simulink library "xrbsDSP_r4"  (Simulink 7.1)
undefined symbols (not defined in the file or in its folder): mem
libraries: xbsIndex_r4 x330
(part 3 of 5)

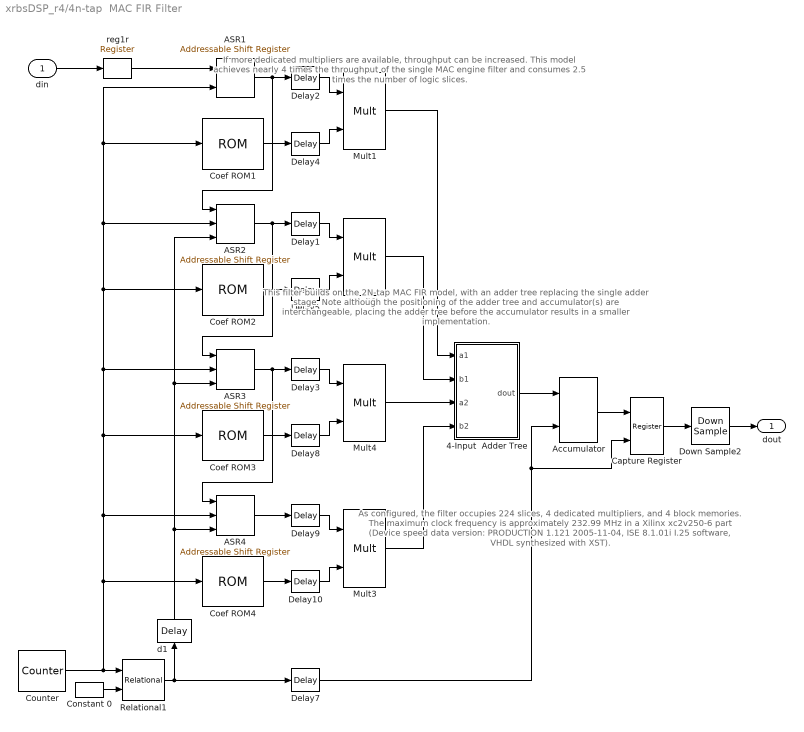
== system xrbsDSP_r4/4n-tap  MAC FIR Filter ==
  note: This filter builds on the 2N-tap MAC FIR model, with an adder tree
      | replacing the single adder stage.  Note although the positioning
      | of the adder tree and accumulator(s) are interchangeable, placing
      | the adder tree before the accumulator results in a smaller
      | implementation.
  note: As configured, the filter occupies 224 slices, 4 dedicated multipliers,
      | and 4 block memories.  The maximum clock frequency is approximately
      |  232.99 MHz in a Xilinx xc2v250-6 part (Device speed data version:
      | PRODUCTION 1.121 2005-11-04, ISE 8.1.01i I.25 software, VHDL
      | synthesized with XST).
  note: If more dedicated multipliers are available, throughput
      | can be increased.  This model achieves nearly 4 times
      | the throughput of the single MAC engine filter and
      | consumes 2.5 times the number of logic slices.
  din : Inport  OutDataType=sfix(16)  OutScaling=2^0
  4-Input  Adder Tree : Subsystem
  ASR1 : xbsIndex_r4/Addressable Shift Register  infer_latency=on  depth=2  initVector=0  en=off  dbl_ovrd=off  use_behavioral_HDL=off  use_rpm=off  block_type=addrsr
      settings: infoedit="Delay of configurable length.  Any element in the delay line can be addressed and driven onto the output port.<P><P>Hardware notes: Implemented using SRL16s.  If a Virtex-II device is used, multiple SRLC16s are cascaded together."  xl_area=[0, 0, 0, 0, 0, 0, 0]  block_version=VER_STRING_GOES_HERE
  ASR2 : xbsIndex_r4/Addressable Shift Register  infer_latency=on  depth=2  initVector=0  en=on  dbl_ovrd=off  use_behavioral_HDL=off  use_rpm=off  block_type=addrsr
      settings: infoedit="Delay of configurable length.  Any element in the delay line can be addressed and driven onto the output port.<P><P>Hardware notes: Implemented using SRL16s.  If a Virtex-II device is used, multiple SRLC16s are cascaded together."  xl_area=[0, 0, 0, 0, 0, 0, 0]  block_version=VER_STRING_GOES_HERE
  ASR3 : xbsIndex_r4/Addressable Shift Register  infer_latency=on  depth=2  initVector=0  en=on  dbl_ovrd=off  use_behavioral_HDL=off  use_rpm=off  block_type=addrsr
      settings: infoedit="Delay of configurable length.  Any element in the delay line can be addressed and driven onto the output port.<P><P>Hardware notes: Implemented using SRL16s.  If a Virtex-II device is used, multiple SRLC16s are cascaded together."  xl_area=[0, 0, 0, 0, 0, 0, 0]  block_version=VER_STRING_GOES_HERE
  ASR4 : xbsIndex_r4/Addressable Shift Register  infer_latency=on  depth=2  initVector=0  en=on  dbl_ovrd=off  use_behavioral_HDL=off  use_rpm=off  block_type=addrsr
      settings: infoedit="Delay of configurable length.  Any element in the delay line can be addressed and driven onto the output port.<P><P>Hardware notes: Implemented using SRL16s.  If a Virtex-II device is used, multiple SRLC16s are cascaded together."  xl_area=[0, 0, 0, 0, 0, 0, 0]  block_version=VER_STRING_GOES_HERE
  Accumulator : xbsIndex_r4/Accumulator  operation=Add  n_bits=ceil(log2(max(1,sum(abs(coef*2^coef_bin_pt)))))+smpl_n_bits + 1  overflow=Wrap  scale=1  rst=on  hasbypass=on  en=off  dbl_ovrd=off  block_type=accum
      settings: infoedit="Adder or subtractor-based accumulator.   Output type and binary point position match the input.<P><P>Hardware notes: When \"Reinitialize with Input 'b' on Reset\" is selected, the accumulator is forced to run at the system rate even if the input 'b' is running at a slower rate."  xl_area=[0, 0, 0, 0, 0, 0, 0]  block_version=VER_STRING_GOES_HERE
  Capture Register : xbsIndex_r4/Register  init=0  rst=off  en=on  dbl_ovrd=off  block_type=register
      settings: xl_area=[0, 0, 0, 0, 0, 0, 0]  block_version=VER_STRING_GOES_HERE
  Coef ROM1 : xbsIndex_r4/ROM  depth=length(coef)/4  initVector=coef(1:(length(coef)/4))  distributed_mem=Block RAM  rst=off  init_reg=0  en=off  latency=1  arith_type="Signed  (2's comp)"  n_bits=coef_n_bits  bin_pt=coef_bin_pt  dbl_ovrd=off  use_rpm=off  block_type=sprom
      settings: xl_area=[0, 0, 0, 0, 0, 0, 0]  block_version=VER_STRING_GOES_HERE
  Coef ROM2 : xbsIndex_r4/ROM  depth=length(coef)/4  initVector=coef((length(coef)/4)+1:length(coef)/2)  distributed_mem=Block RAM  rst=off  init_reg=0  en=off  latency=1  arith_type="Signed  (2's comp)"  n_bits=coef_n_bits  bin_pt=coef_bin_pt  dbl_ovrd=off  use_rpm=off  block_type=sprom
      settings: xl_area=[0, 0, 0, 0, 0, 0, 0]  block_version=VER_STRING_GOES_HERE
  Coef ROM3 : xbsIndex_r4/ROM  depth=length(coef)/4  initVector=coef((length(coef)/2)+1:(3/4)*length(coef))  distributed_mem=Block RAM  rst=off  init_reg=0  en=off  latency=1  arith_type="Signed  (2's comp)"  n_bits=coef_n_bits  bin_pt=coef_bin_pt  dbl_ovrd=off  use_rpm=off  block_type=sprom
      settings: xl_area=[0, 0, 0, 0, 0, 0, 0]  block_version=VER_STRING_GOES_HERE
  Coef ROM4 : xbsIndex_r4/ROM  depth=length(coef)/4  initVector=coef((3/4)*length(coef)+1:length(coef))  distributed_mem=Block RAM  rst=off  init_reg=0  en=off  latency=1  arith_type="Signed  (2's comp)"  n_bits=coef_n_bits  bin_pt=coef_bin_pt  dbl_ovrd=off  use_rpm=off  block_type=sprom
      settings: xl_area=[0, 0, 0, 0, 0, 0, 0]  block_version=VER_STRING_GOES_HERE
  Constant 0 : xbsIndex_r4/Constant  arith_type=Unsigned  const=0  n_bits=1  bin_pt=0  explicit_period=off  period=1  equ=P=C  opselect=C  inp2=PCIN>>17  opr=+  inp1=P  carry=CIN  dbl_ovrd=off  block_type=constant
      settings: block_version=VER_STRING_GOES_HERE
  Counter : xbsIndex_r4/Counter  cnt_type=Count Limited  cnt_to=(length(coef)/4)-1  operation=Up  start_count=0  cnt_by_val=1  arith_type=Unsigned  n_bits=ceil(log2(length(coef)/4))  bin_pt=0  load_pin=off  rst=off  en=off  dbl_ovrd=off  explicit_period=on  period=smpl_period/(length(coef)/4)  block_type=counter
      settings: infoedit="Configurable up, down and up/down counter.<P><P>Hardware notes: Free running counters are the least expensive in hardware.  A count limited counter is implemented by combining a counter with a comparator."  xl_area=[0, 0, 0, 0, 0, 0, 0]  block_version=VER_STRING_GOES_HERE
  Delay{1..3,9} (4 alike) : xbsIndex_r4/Delay  en=off  latency=2  dbl_ovrd=off  reg_retiming=off  block_type=delay
      settings: infoedit="Delay line having  configurable length.<P><P>Hardware notes: A delay line is a chain, each link of which is an SRL16 followed by a flip-flop. If register retiming is enabled, the delay line is a chain of flip-flops."  xl_area=[0, 0, 0, 0, 0, 0, 0]  block_version=VER_STRING_GOES_HERE
  Delay{4..5,8,10} (4 alike) : xbsIndex_r4/Delay  en=off  latency=1  dbl_ovrd=off  reg_retiming=off  block_type=delay
      settings: infoedit="Delay line having  configurable length.<P><P>Hardware notes: A delay line is a chain, each link of which is an SRL16 followed by a flip-flop. If register retiming is enabled, the delay line is a chain of flip-flops."  xl_area=[0, 0, 0, 0, 0, 0, 0]  block_version=VER_STRING_GOES_HERE
  Delay7 : xbsIndex_r4/Delay  en=off  latency=5  dbl_ovrd=off  reg_retiming=off  block_type=delay
      settings: infoedit="Delay line having  configurable length.<P><P>Hardware notes: A delay line is a chain, each link of which is an SRL16 followed by a flip-flop. If register retiming is enabled, the delay line is a chain of flip-flops."  xl_area=[0, 0, 0, 0, 0, 0, 0]  block_version=VER_STRING_GOES_HERE
  Down Sample2 : xbsIndex_r4/Down Sample  sample_ratio=length(coef)/4  sample_phase="Last Value of Frame  (most efficient)"  en=off  latency=1  dbl_ovrd=off  block_type=dsamp
      settings: xl_area=[0, 0, 0, 0, 0, 0, 0]  block_version=VER_STRING_GOES_HERE
  Mult{1..4} (4 alike) : xbsIndex_r4/Mult  precision=User Defined  arith_type="Signed  (2's comp)"  n_bits=max(ceil(log2(max(1,max(abs(coef*2^coef_bin_pt)))))+smpl_n_bits + 1,smpl_bin_pt+coef_bin_pt)  bin_pt=smpl_bin_pt+coef_bin_pt  quantization=Truncate  overflow=Wrap  en=off  latency=2  dbl_ovrd=off  use_behavioral_HDL=off  use_embedded=on  pipeline=on  use_rpm=on  placement_style=Rectangular shape  block_type=mult
      settings: infoedit=Multiplies two values.<P><P>Hardware notes: To use the internal pipeline stage of the dedicated multiplier you must select 'Pipeline to Greatest Extent Possible'.  xl_area=[0, 0, 0, 0, 0, 0, 0]  block_version=VER_STRING_GOES_HERE
  Relational1 : xbsIndex_r4/Relational  mode=a=b  en=off  latency=1  dbl_ovrd=off  block_type=relational
      settings: xl_area=[0, 0, 0, 0, 0, 0, 0]  block_version=VER_STRING_GOES_HERE
  d1 : xbsIndex_r4/Delay  Orientation=up  en=off  latency=(length(coef)/4)-2  dbl_ovrd=off  reg_retiming=off  block_type=delay
      settings: infoedit="Delay line having  configurable length.<P><P>Hardware notes: A delay line is a chain, each link of which is an SRL16 followed by a flip-flop. If register retiming is enabled, the delay line is a chain of flip-flops."  xl_area=[0, 0, 0, 0, 0, 0, 0]  block_version=VER_STRING_GOES_HERE
  reg1r : xbsIndex_r4/Register  init=0  rst=off  en=off  dbl_ovrd=off  block_type=register
      settings: xl_area=[0, 0, 0, 0, 0, 0, 0]  block_version=VER_STRING_GOES_HERE
  dout : Outport  OutDataType=sfix(16)  OutScaling=2^0
  wires:
  Constant 0/1 -> Relational1/2
  din/1 -> reg1r/1
  reg1r/1 -> ASR1/1
  Coef ROM1/1 -> Delay4/1
  ASR1/1 -> Delay2/1, ASR2/1
  Coef ROM2/1 -> Delay5/1
  ASR2/1 -> Delay1/1, ASR3/1
  Delay2/1 -> Mult1/1
  Delay1/1 -> Mult2/1
  Mult1/1 -> 4-Input  Adder Tree/1(a1)
  Mult2/1 -> 4-Input  Adder Tree/2(b1)
  Counter/1 -> Relational1/1, ASR4/2, Coef ROM3/1, ASR3/2, Coef ROM2/1, ASR2/2, ASR1/2, Coef ROM1/1, Coef ROM4/1
  Relational1/1 -> d1/1, Delay7/1
  Coef ROM3/1 -> Delay8/1
  ASR3/1 -> Delay3/1, ASR4/1
  Delay3/1 -> Mult4/1
  Coef ROM4/1 -> Delay10/1
  ASR4/1 -> Delay9/1
  Delay9/1 -> Mult3/1
  Mult3/1 -> 4-Input  Adder Tree/4(b2)
  Delay5/1 -> Mult2/2
  Delay8/1 -> Mult4/2
  Delay4/1 -> Mult1/2
  Delay10/1 -> Mult3/2
  d1/1 -> ASR4/3, ASR2/3, ASR3/3
  Accumulator/1 -> Capture Register/1
  Capture Register/1 -> Down Sample2/1
  Down Sample2/1 -> dout/1
  Mult4/1 -> 4-Input  Adder Tree/3(a2)
  4-Input  Adder Tree/1(dout) -> Accumulator/1
  Delay7/1 -> Accumulator/2, Capture Register/2

== system xrbsDSP_r4/CIC Filter ==
  note: The Interpoiation by 48, 4 stage CIC filter occupies 116 slices.
      | The maximum clock frequency is approximately
      | 308.55 MHz in a Xilinx xc2vp2-7 part (Device speed data version:
      | PRODUCTION 1.121 2005-11-04, ISE 8.1.01i I.25 software, VHDL
      | synthesized with XST).
  note: The CIC filter is constructed out of differentiators and integrators and
      | a sample rate change. This block provides a full precision result and is
      | dynamically built given the parameters entered in the dialog box. The
      | dynamic rebuilding script can switch which side the integrators and
      | differentiators are on and also change between an up and down sampler
      | depending on whether an Interpolator or decimator is selected respectively.
      | The number of stages selected control how many integrators and
      | differentiators are used.
  In1 : Inport  OutDataType=sfix(16)  OutScaling=2^0
  Differentiator1 : Subsystem  mask(Differentiator Stage){m=m, output_bitwidth=ceil(stages*log2(rate_change*m) + input_bitwidth), output_binpt=input_binpt}
      mask prompts: m "Differential Delay"; output_bitwidth "Output Bit Width"; output_binpt "Output Binary Point"
      mask help: Multi-Channel Differentiator
      mask init:
      | set_param(gcb, 'LinkStatus', 'none');
  Differentiator2 : Subsystem  mask(Differentiator Stage){m=m, output_bitwidth=ceil(stages*log2(rate_change*m) + input_bitwidth), output_binpt=input_binpt}
      mask prompts: m "Differential Delay"; output_bitwidth "Output Bit Width"; output_binpt "Output Binary Point"
      mask help: Multi-Channel Differentiator
      mask init:
      | set_param(gcb, 'LinkStatus', 'none');
  Differentiator3 : Subsystem  mask(Differentiator Stage){m=m, output_bitwidth=ceil(stages*log2(rate_change*m) + input_bitwidth), output_binpt=input_binpt}
      mask prompts: m "Differential Delay"; output_bitwidth "Output Bit Width"; output_binpt "Output Binary Point"
      mask help: Multi-Channel Differentiator
      mask init:
      | set_param(gcb, 'LinkStatus', 'none');
  Down Sample : xbsIndex_r4/Down Sample  sample_ratio=rate_change  sample_phase=First Value of Frame  en=off  latency=1  dbl_ovrd=off  block_type=dsamp
      settings: block_version=9.2.00
  Integrator1 : Subsystem  mask(Integrator Stage){output_bitwidth=ceil(stages*log2(rate_change*m) + input_bitwidth)}
      mask prompts: output_bitwidth "Output Bit Width"
      mask help: Multi Channel Integrator
      mask init:
      | set_param(gcb, 'LinkStatus', 'none');
      settings: CopyFcn=set_param(gcb, 'LinkStatus', 'none');
  Integrator2 : Subsystem  mask(Integrator Stage){output_bitwidth=ceil(stages*log2(rate_change*m) + input_bitwidth)}
      mask prompts: output_bitwidth "Output Bit Width"
      mask help: Multi Channel Integrator
      mask init:
      | set_param(gcb, 'LinkStatus', 'none');
      settings: CopyFcn=set_param(gcb, 'LinkStatus', 'none');
  Integrator3 : Subsystem  mask(Integrator Stage){output_bitwidth=ceil(stages*log2(rate_change*m) + input_bitwidth)}
      mask prompts: output_bitwidth "Output Bit Width"
      mask help: Multi Channel Integrator
      mask init:
      | set_param(gcb, 'LinkStatus', 'none');
      settings: CopyFcn=set_param(gcb, 'LinkStatus', 'none');
  Out1 : Outport  OutDataType=sfix(16)  OutScaling=2^0
  wires:
  Differentiator3/1(Out1) -> Out1/1
  Integrator3/1(Out1) -> Down Sample/1
  Differentiator2/1(Out1) -> Differentiator3/1(In1)
  Integrator2/1(Out1) -> Integrator3/1(In1)
  Differentiator1/1(Out1) -> Differentiator2/1(In1)
  Integrator1/1(Out1) -> Integrator2/1(In1)
  Down Sample/1 -> Differentiator1/1(In1)
  In1/1 -> Integrator1/1(In1)

== system xrbsDSP_r4/Dual Port Memory Interpolation MAC FIR Filter ==
  note: The control logic provides the
      | necessary address logic for the
      | Dual Port RAM. The control logic
      | creates a cyclic RAM buffer for
      | port A (data buffer) to create the
      | shifting effect required.
  note: A 'Dual Port Block RAM' subystem implements the
      | input data buffer.  The address port runs n times
      | faster than the data port, where n is the number
      | of filter taps.
      |
      | The filter coefficients are also stored in the same
      | Dual Port Block RAM and are output from port B.
  note: As configured, the filter occupies 117 slices, 1 dedicated
      | multiplier, and 1 block memory. The maximum clock
      | frequency is approximately 268.89 MHz in a Xilinx
      | xc2vp2-7 part (Device speed data version: PRODUCTION
      | 1.121 2005-11-04, ISE 8.1.01i I.25 software, VHDL
      | synthesized with XST).
  note: A capture register is required for streaming
      | operation, since the MAC engine reloads its
      | accumulator with an incoming sample after
      | computing the last partial product for an output
      | sample.
  note: A down sampler reduces the capture register
      | sample period to the output sample period. Note that
      | the down sample is less than the up sample to achieve
      | the correct interpolation rate.
      |
      | The block is configured with latency to obtain  the
      | most efficient hardware implementation.  The down
      | sampling rate is equal to the coefficient array length.
  Din : Inport  OutDataType=sfix(16)  OutScaling=2^0
  Accumulator : xbsIndex_r4/Accumulator  operation=Add  n_bits=accum_bit_width  overflow=Wrap  scale=1  rst=on  hasbypass=on  en=off  dbl_ovrd=off  block_type=accum
      settings: infoedit="Adder or subtractor-based accumulator.   Output type and binary point position match the input.<P><P>Hardware notes: When \"Reinitialize with Input 'b' on Reset\" is selected, the accumulator is forced to run at the system rate even if the input 'b' is running at a slower rate."  xl_area=[18 36 0 36 0 0 0]  block_version=VER_STRING_GOES_HERE
  Address Control : Subsystem
  Delay2 : xbsIndex_r4/Delay  en=off  latency=4  dbl_ovrd=off  reg_retiming=off  block_type=delay
      settings: infoedit="Delay line having  configurable length.<P><P>Hardware notes: A delay line is a chain, each link of which is an SRL16 followed by a flip-flop. If register retiming is enabled, the delay line is a chain of flip-flops."  xl_area=[1 1 0 1 0 0 0]  block_version=VER_STRING_GOES_HERE
  Down Sample : xbsIndex_r4/Down Sample  sample_ratio=length(coef)/ir  sample_phase="Last Value of Frame  (most efficient)"  en=off  latency=1  dbl_ovrd=off  block_type=dsamp
      settings: xl_area=[18 36 0 0 0 0 0]  block_version=VER_STRING_GOES_HERE
  Dual Port RAM : Subsystem
  Mult : xbsIndex_r4/Mult  precision=Full  arith_type="Signed  (2's comp)"  n_bits=8  bin_pt=2  quantization=Truncate  overflow=Wrap  en=off  latency=2  dbl_ovrd=off  use_behavioral_HDL=off  use_embedded=on  pipeline=on  use_rpm=off  placement_style=Rectangular shape  block_type=mult
      settings: infoedit=Multiplies two values.<P><P>Hardware notes: To use the internal pipeline stage of the dedicated multiplier you must select 'Pipeline to Greatest Extent Possible'.  xl_area=[18 36 0 0 0 1 0]  block_version=VER_STRING_GOES_HERE
  Register : xbsIndex_r4/Register  init=0  rst=off  en=on  dbl_ovrd=off  block_type=register
      settings: xl_area=[18 36 0 0 0 0 0]  block_version=VER_STRING_GOES_HERE
  Dout : Outport  OutDataType=sfix(16)  OutScaling=2^0
  wires:
  Delay2/1 -> Register/2, Accumulator/2
  Address Control/4(reset) -> Delay2/1
  Dual Port RAM/2(dout_B) -> Mult/2
  Dual Port RAM/1(dout_A) -> Mult/1
  Din/1 -> Dual Port RAM/1(data_A)
  Address Control/3(coef_addr) -> Dual Port RAM/4(addr_B)
  Address Control/2(we) -> Dual Port RAM/3(we_A)
  Address Control/1(data_addr) -> Dual Port RAM/2(addr_A)
  Register/1 -> Down Sample/1
  Accumulator/1 -> Register/1
  Down Sample/1 -> Dout/1
  Mult/1 -> Accumulator/1

== system xrbsDSP_r4/Interpolation Filter ==
  note: The coefficients are arranged in
      | the memory in phase filter order
      | as each phase filter of the polyphase
      | structure is calculated in sequence.
      | The coefficients are pre-arranged by
      | the mask of this block and stored
      | in the appropritate memories
  note: The down sampler is smaller
      | than the initial upsample to
      | achieve the appropriate
      | interpolated rate
  note: The accumulator sums up
      | the partial products from the
      | mult adder tree to form the
      | complete result from each phase
      | filter of the polyphase arms
  note: The 'Adder Tree' subsystem
      | sums the multiplication
      | results after they are
      | caluculated
  note: The 'Multipliers' subsystem
      | employs 4 multiplier to
      | calculate the coefficient
      | and data products.  Data
      | and coefficients are changed
      | to complete the result
  note: As configured, the filter occupies 142 slices, 4 dedicated multipliers, and
      | 4 block memory.  The maximum clock frequency is approximately
      | 269.76 MHz in a Xilinx xc2vp2-7 part (Device speed data version:
      | PRODUCTION 1.121 2005-11-04, ISE 8.1.01i I.25 software, VHDL
      | synthesized with XST).
  din : Inport  OutDataType=sfix(16)  OutScaling=2^0
  Accumulator : xbsIndex_r4/Accumulator  operation=Add  n_bits=y_bit_width  overflow=Wrap  scale=1  rst=on  hasbypass=on  en=off  dbl_ovrd=off  block_type=accum
      settings: infoedit="Adder or subtractor-based accumulator.   Output type and binary point position match the input.<P><P>Hardware notes: When \"Reinitialize with Input 'b' on Reset\" is selected, the accumulator is forced to run at the system rate even if the input 'b' is running at a slower rate."  xl_area=[0, 0, 0, 0, 0, 0, 0]  block_version=VER_STRING_GOES_HERE
  Adder Tree : Subsystem
  Coef Buffer : Subsystem
  Control : Subsystem
  Data Buffer : Subsystem
  Delay : xbsIndex_r4/Delay  en=off  latency=5  dbl_ovrd=off  reg_retiming=off  block_type=delay
      settings: infoedit="Delay line having  configurable length.<P><P>Hardware notes: A delay line is a chain, each link of which is an SRL16 followed by a flip-flop. If register retiming is enabled, the delay line is a chain of flip-flops."  xl_area=[0, 0, 0, 0, 0, 0, 0]  block_version=VER_STRING_GOES_HERE
  Delay2 : xbsIndex_r4/Delay  en=on  latency=1  dbl_ovrd=off  reg_retiming=off  block_type=delay
      settings: infoedit="Delay line having  configurable length.<P><P>Hardware notes: A delay line is a chain, each link of which is an SRL16 followed by a flip-flop. If register retiming is enabled, the delay line is a chain of flip-flops."  xl_area=[0, 0, 0, 0, 0, 0, 0]  block_version=VER_STRING_GOES_HERE
  Down Sample : xbsIndex_r4/Down Sample  sample_ratio=downsamp_by  sample_phase="Last Value of Frame  (most efficient)"  en=off  latency=1  dbl_ovrd=off  block_type=dsamp
      settings: xl_area=[0, 0, 0, 0, 0, 0, 0]  block_version=VER_STRING_GOES_HERE
  Mutlipliers : Subsystem
  Up Sample : xbsIndex_r4/Up Sample  sample_ratio=upsamp_by  copy_samples=on  dbl_ovrd=off  block_type=usamp
      settings: infoedit="Up samples input data.  Inserted values  can be zeros or copies of the most recent input sample.<P><P>Hardware notes: No hardware is needed if inserted values are copies of the input sample; otherwise, a mux and single bit flip-flop are used."  xl_area=[0, 0, 0, 0, 0, 0, 0]  block_version=VER_STRING_GOES_HERE
  Out1 : Outport  OutDataType=sfix(16)  OutScaling=2^0
  wires:
  Delay2/1 -> Down Sample/1
  Accumulator/1 -> Delay2/1
  Down Sample/1 -> Out1/1
  din/1 -> Up Sample/1
  Adder Tree/1(sum) -> Accumulator/1
  Mutlipliers/4(p3) -> Adder Tree/4(din4)
  Mutlipliers/3(p2) -> Adder Tree/3(din3)
  Mutlipliers/2(p1) -> Adder Tree/2(din2)
  Mutlipliers/1(p0) -> Adder Tree/1(din1)
  Delay/1 -> Delay2/2, Accumulator/2
  Coef Buffer/4(coef3) -> Mutlipliers/8(b3)
  Coef Buffer/3(coef2) -> Mutlipliers/6(b2)
  Coef Buffer/2(coef1) -> Mutlipliers/4(b1)
  Coef Buffer/1(coef0) -> Mutlipliers/2(b0)
  Data Buffer/4(data3) -> Mutlipliers/7(a3)
  Data Buffer/3(data2) -> Mutlipliers/5(a2)
  Data Buffer/2(data1) -> Mutlipliers/3(a1)
  Data Buffer/1(data0) -> Mutlipliers/1(a0)
  Control/4(srl16_we) -> Delay/1
  Control/3(coef_addr) -> Coef Buffer/1(addr)
  Control/2(result) -> Data Buffer/3(shift_en)
  Control/1(data_addr) -> Data Buffer/2(addr)
  Up Sample/1 -> Data Buffer/1(din)

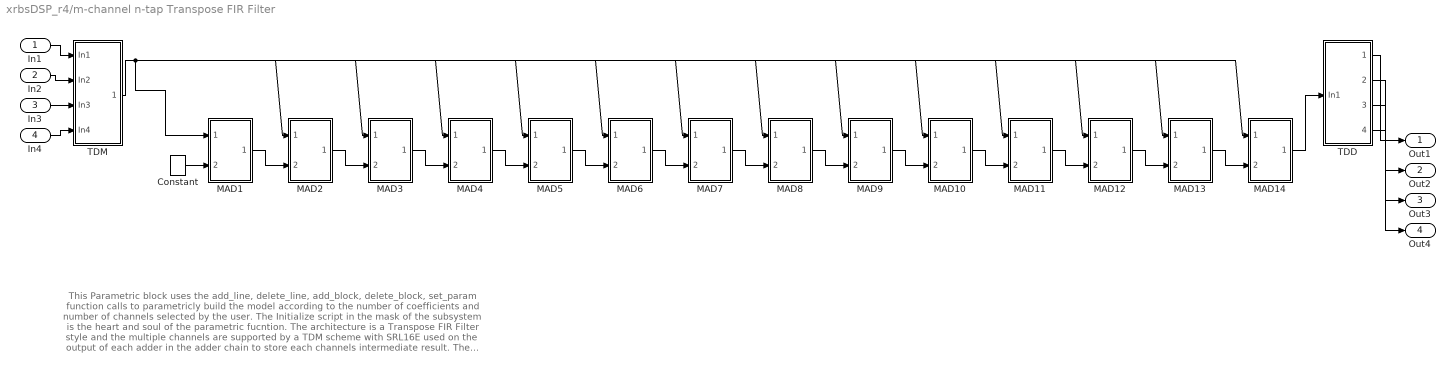
== system xrbsDSP_r4/m-channel n-tap Transpose FIR Filter ==
  note: This Parametric block uses the add_line, delete_line, add_block, delete_block, set_param function calls to parametricly
      | build the model according to the number of coefficients and number of channels selected by the user. The Initialize script in
      | the mask of the subsystem is the heart and soul of the parametric fucntion.
      |
      | The architecture is a Transpose FIR Filter style and the multiple channels are supported by a TDM scheme with SRL16E used
      | on the output of each adder in the adder chain to store each channels intermediate result. The clock will always be N channels
      | times faster that the input sample rate.
  In1 : Inport  OutDataType=sfix(16)  OutScaling=2^0
  In2 : Inport  Port=2  OutDataType=sfix(16)  OutScaling=2^0
  In3 : Inport  Port=3  OutDataType=sfix(16)  OutScaling=2^0
  In4 : Inport  Port=4  OutDataType=sfix(16)  OutScaling=2^0
  Constant : xbsIndex_r4/Constant  arith_type=Unsigned  const=0  n_bits=1  bin_pt=0  explicit_period=off  period=1  equ=P=C  opselect=C  inp2=PCIN>>17  opr=+  inp1=P  carry=CIN  dbl_ovrd=off  block_type=constant
      settings: block_version=VER_STRING_GOES_HERE
  MAD1 : Subsystem  mask(MAD Block){coef=coef_array(1), coef_bitwidth=coef_bitwidth, coef_binpt=coef_binpt, channels=channels}
      mask prompts: coef "Coefficient Value"; coef_bitwidth "Coefficient Bit Width"; coef_binpt "Coefficient Binary Point"; channels "Number of Channels"
  MAD10 : Subsystem  mask(MAD Block){coef=coef_array(10), coef_bitwidth=coef_bitwidth, coef_binpt=coef_binpt, channels=channels}
      mask prompts: coef "Coefficient Value"; coef_bitwidth "Coefficient Bit Width"; coef_binpt "Coefficient Binary Point"; channels "Number of Channels"
  MAD11 : Subsystem  mask(MAD Block){coef=coef_array(11), coef_bitwidth=coef_bitwidth, coef_binpt=coef_binpt, channels=channels}
      mask prompts: coef "Coefficient Value"; coef_bitwidth "Coefficient Bit Width"; coef_binpt "Coefficient Binary Point"; channels "Number of Channels"
  MAD12 : Subsystem  mask(MAD Block){coef=coef_array(12), coef_bitwidth=coef_bitwidth, coef_binpt=coef_binpt, channels=channels}
      mask prompts: coef "Coefficient Value"; coef_bitwidth "Coefficient Bit Width"; coef_binpt "Coefficient Binary Point"; channels "Number of Channels"
  MAD13 : Subsystem  mask(MAD Block){coef=coef_array(13), coef_bitwidth=coef_bitwidth, coef_binpt=coef_binpt, channels=channels}
      mask prompts: coef "Coefficient Value"; coef_bitwidth "Coefficient Bit Width"; coef_binpt "Coefficient Binary Point"; channels "Number of Channels"
  MAD14 : Subsystem  mask(MAD Block){coef=coef_array(14), coef_bitwidth=coef_bitwidth, coef_binpt=coef_binpt, channels=channels}
      mask prompts: coef "Coefficient Value"; coef_bitwidth "Coefficient Bit Width"; coef_binpt "Coefficient Binary Point"; channels "Number of Channels"
  MAD2 : Subsystem  mask(MAD Block){coef=coef_array(2), coef_bitwidth=coef_bitwidth, coef_binpt=coef_binpt, channels=channels}
      mask prompts: coef "Coefficient Value"; coef_bitwidth "Coefficient Bit Width"; coef_binpt "Coefficient Binary Point"; channels "Number of Channels"
  MAD3 : Subsystem  mask(MAD Block){coef=coef_array(3), coef_bitwidth=coef_bitwidth, coef_binpt=coef_binpt, channels=channels}
      mask prompts: coef "Coefficient Value"; coef_bitwidth "Coefficient Bit Width"; coef_binpt "Coefficient Binary Point"; channels "Number of Channels"
  MAD4 : Subsystem  mask(MAD Block){coef=coef_array(4), coef_bitwidth=coef_bitwidth, coef_binpt=coef_binpt, channels=channels}
      mask prompts: coef "Coefficient Value"; coef_bitwidth "Coefficient Bit Width"; coef_binpt "Coefficient Binary Point"; channels "Number of Channels"
  MAD5 : Subsystem  mask(MAD Block){coef=coef_array(5), coef_bitwidth=coef_bitwidth, coef_binpt=coef_binpt, channels=channels}
      mask prompts: coef "Coefficient Value"; coef_bitwidth "Coefficient Bit Width"; coef_binpt "Coefficient Binary Point"; channels "Number of Channels"
  MAD6 : Subsystem  mask(MAD Block){coef=coef_array(6), coef_bitwidth=coef_bitwidth, coef_binpt=coef_binpt, channels=channels}
      mask prompts: coef "Coefficient Value"; coef_bitwidth "Coefficient Bit Width"; coef_binpt "Coefficient Binary Point"; channels "Number of Channels"
  MAD7 : Subsystem  mask(MAD Block){coef=coef_array(7), coef_bitwidth=coef_bitwidth, coef_binpt=coef_binpt, channels=channels}
      mask prompts: coef "Coefficient Value"; coef_bitwidth "Coefficient Bit Width"; coef_binpt "Coefficient Binary Point"; channels "Number of Channels"
  MAD8 : Subsystem  mask(MAD Block){coef=coef_array(8), coef_bitwidth=coef_bitwidth, coef_binpt=coef_binpt, channels=channels}
      mask prompts: coef "Coefficient Value"; coef_bitwidth "Coefficient Bit Width"; coef_binpt "Coefficient Binary Point"; channels "Number of Channels"
  MAD9 : Subsystem  mask(MAD Block){coef=coef_array(9), coef_bitwidth=coef_bitwidth, coef_binpt=coef_binpt, channels=channels}
      mask prompts: coef "Coefficient Value"; coef_bitwidth "Coefficient Bit Width"; coef_binpt "Coefficient Binary Point"; channels "Number of Channels"
  TDD : Subsystem
      mask Type: TDD
      mask Description: Multi-Channel Time Division DeMultiplexer
  TDM : Subsystem
  Out1 : Outport  OutDataType=sfix(16)  OutScaling=2^0
  Out2 : Outport  Port=2  OutDataType=sfix(16)  OutScaling=2^0
  Out3 : Outport  Port=3  OutDataType=sfix(16)  OutScaling=2^0
  Out4 : Outport  Port=4  OutDataType=sfix(16)  OutScaling=2^0
  wires:
  MAD14/1(Out1) -> TDD/1(In1)
  MAD13/1(Out1) -> MAD14/2(In2)
  MAD12/1(Out1) -> MAD13/2(In2)
  MAD11/1(Out1) -> MAD12/2(In2)
  MAD10/1(Out1) -> MAD11/2(In2)
  MAD9/1(Out1) -> MAD10/2(In2)
  MAD8/1(Out1) -> MAD9/2(In2)
  MAD7/1(Out1) -> MAD8/2(In2)
  MAD6/1(Out1) -> MAD7/2(In2)
  MAD5/1(Out1) -> MAD6/2(In2)
  MAD4/1(Out1) -> MAD5/2(In2)
  MAD3/1(Out1) -> MAD4/2(In2)
  MAD2/1(Out1) -> MAD3/2(In2)
  MAD1/1(Out1) -> MAD2/2(In2)
  TDM/1(Out1) -> MAD14/1(In1), MAD13/1(In1), MAD12/1(In1), MAD11/1(In1), MAD10/1(In1), MAD9/1(In1), MAD8/1(In1), MAD7/1(In1), MAD6/1(In1), MAD5/1(In1), MAD4/1(In1), MAD3/1(In1), MAD2/1(In1), MAD1/1(In1)
  Constant/1 -> MAD1/2(In2)
  In1/1 -> TDM/1(In1)
  TDD/1(Out1) -> Out1/1
  In2/1 -> TDM/2(In2)
  In3/1 -> TDM/3(In3)
  In4/1 -> TDM/4(In4)
  TDD/2(Out2) -> Out2/1
  TDD/3(Out3) -> Out3/1
  TDD/4(Out4) -> Out4/1

== system xrbsDSP_r4/n-tap Dual Port Memory MAC FIR Filter ==
  note: The 'Address Control' subsystem
      | provides the necessary address
      | logic for the Dual Port RAM.
      | The control logic creates a cyclic
      | RAM buffer for port A (data buffer)
      | to create the required shifting
      | effect.
  note: A Dual Port Block RAM implements the input data buffer.
      | The address port runs n times faster than the data port,
      | where n is the number of filter taps.
      |
      | The filter coefficients are also stored in the same Dual Port
      | Block RAM and are output from port B.
  note: A down sampler reduces the capture register
      | sample period to the output sample period.
      | The block is configured with latency to obtain  the
      | most efficient hardware implementation.  The down
      | sampling rate is equal to the coefficient array length.
  note: A capture register is required for streaming
      | operation, since the MAC engine reloads its
      | accumulator with an incoming sample after
      | computing the last partial product for an output
      | sample.
  note: As configured, the filter occupies 95 slices, 1 dedicated multiplier,
      | and 1 block memory.  The maximum clock frequency is approximately
      | 279.41 MHz in a Xilinx xc2vp2-7 part (Device speed data version:
      | PRODUCTION 1.121 2005-11-04, ISE 8.1.01i I.25 software, VHDL
      | synthesized with XST).
  din : Inport  OutDataType=sfix(16)  OutScaling=2^0
  Accumulator : xbsIndex_r4/Accumulator  operation=Add  n_bits=accum_bit_width  overflow=Wrap  scale=1  rst=on  hasbypass=on  en=off  dbl_ovrd=off  block_type=accum
      settings: infoedit="Adder or subtractor-based accumulator.   Output type and binary point position match the input.<P><P>Hardware notes: When \"Reinitialize with Input 'b' on Reset\" is selected, the accumulator is forced to run at the system rate even if the input 'b' is running at a slower rate."  xl_area=[0, 0, 0, 0, 0, 0, 0]  block_version=VER_STRING_GOES_HERE
  Address Control : Subsystem
  Capture Register : xbsIndex_r4/Register  init=0  rst=off  en=on  dbl_ovrd=off  block_type=register
      settings: xl_area=[0, 0, 0, 0, 0, 0, 0]  block_version=VER_STRING_GOES_HERE
  Delay : xbsIndex_r4/Delay  en=off  latency=3  dbl_ovrd=off  reg_retiming=off  block_type=delay
      settings: infoedit="Delay line having  configurable length.<P><P>Hardware notes: A delay line is a chain, each link of which is an SRL16 followed by a flip-flop. If register retiming is enabled, the delay line is a chain of flip-flops."  xl_area=[0, 0, 0, 0, 0, 0, 0]  block_version=VER_STRING_GOES_HERE
  Down Sample : xbsIndex_r4/Down Sample  sample_ratio=length(coef)  sample_phase="Last Value of Frame  (most efficient)"  en=off  latency=1  dbl_ovrd=off  block_type=dsamp
      settings: xl_area=[0, 0, 0, 0, 0, 0, 0]  block_version=VER_STRING_GOES_HERE
  Dual Port RAM : Subsystem
  Mult : xbsIndex_r4/Mult  precision=Full  arith_type="Signed  (2's comp)"  n_bits=8  bin_pt=2  quantization=Truncate  overflow=Wrap  en=off  latency=2  dbl_ovrd=off  use_behavioral_HDL=off  use_embedded=on  pipeline=on  use_rpm=off  placement_style=Rectangular shape  block_type=mult
      settings: infoedit=Multiplies two values.<P><P>Hardware notes: To use the internal pipeline stage of the dedicated multiplier you must select 'Pipeline to Greatest Extent Possible'.  xl_area=[0, 0, 0, 0, 0, 0, 0]  block_version=VER_STRING_GOES_HERE
  dout : Outport  OutDataType=sfix(16)  OutScaling=2^0
  wires:
  Delay/1 -> Accumulator/2, Capture Register/2
  Address Control/4(rst) -> Delay/1
  Dual Port RAM/2(dout_b) -> Mult/2
  Dual Port RAM/1(dout_a) -> Mult/1
  din/1 -> Dual Port RAM/1(din)
  Address Control/3(coef_addr) -> Dual Port RAM/4(coef_addr)
  Address Control/2(we) -> Dual Port RAM/3(we)
  Address Control/1(data_addr) -> Dual Port RAM/2(data_addr)
  Capture Register/1 -> Down Sample/1
  Accumulator/1 -> Capture Register/1
  Down Sample/1 -> dout/1
  Mult/1 -> Accumulator/1

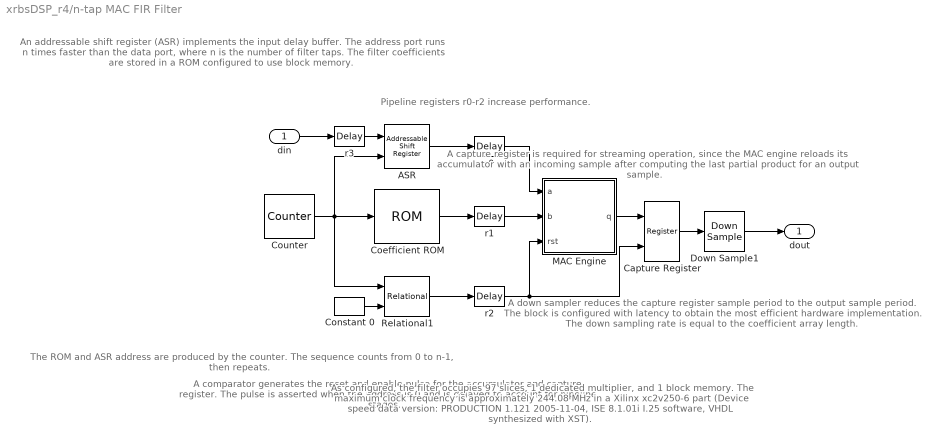
== system xrbsDSP_r4/n-tap MAC FIR Filter ==
  note: A capture register is required for streaming
      | operation, since the MAC engine reloads its
      | accumulator with an incoming sample after
      | computing the last partial product for an output
      | sample.
  note: Pipeline registers r0-r2
      | increase performance.
  note: An addressable shift register (ASR)
      | implements the input delay buffer.
      | The address port runs n times faster
      | than the data port, where n is the number
      | of filter taps.
      |
      | The filter coefficients are stored in a ROM
      | configured to use block memory.
  note: The ROM and ASR
      | address are produced
      | by the counter.  The
      | sequence counts from
      | 0 to n-1, then repeats.
  note: A comparator generates
      | the reset and enable
      | pulse for the accumulator
      | and capture register.  The
      | pulse is asserted when
      | the address is 0 and is
      | delayed to account for
      | pipeline stages.
  note: As configured, the  filter occupies 97 slices, 1 dedicated multiplier, and
      | 1 block memory.  The maximum clock frequency is approximately
      | 244.08 MHz in a Xilinx xc2v250-6 part (Device speed data version:
      | PRODUCTION 1.121 2005-11-04, ISE 8.1.01i I.25 software, VHDL
      | synthesized with XST).
  note: A down sampler reduces the capture register
      | sample period to the output sample period.
      | The block is configured with latency to obtain  the
      | most efficient hardware implementation.  The down
      | sampling rate is equal to the coefficient array length.
  din : Inport  OutDataType=sfix(16)  OutScaling=2^0
  ASR : xbsIndex_r4/Addressable Shift Register  infer_latency=on  depth=2  initVector=0  en=off  dbl_ovrd=off  use_behavioral_HDL=off  use_rpm=off  block_type=addrsr
      settings: infoedit="Delay of configurable length.  Any element in the delay line can be addressed and driven onto the output port.<P><P>Hardware notes: Implemented using SRL16s.  If a Virtex-II device is used, multiple SRLC16s are cascaded together."  xl_area=[0, 0, 0, 0, 0, 0, 0]  block_version=VER_STRING_GOES_HERE
  Capture Register : xbsIndex_r4/Register  init=0  rst=off  en=on  dbl_ovrd=off  block_type=register
      settings: xl_area=[0, 0, 0, 0, 0, 0, 0]  block_version=VER_STRING_GOES_HERE
  Coefficient ROM : xbsIndex_r4/ROM  depth=length(coef)  initVector=coef  distributed_mem=Block RAM  rst=off  init_reg=0  en=off  latency=1  arith_type="Signed  (2's comp)"  n_bits=coef_n_bits  bin_pt=coef_bin_pt  dbl_ovrd=off  use_rpm=off  block_type=sprom
      settings: xl_area=[0, 0, 0, 0, 0, 0, 0]  block_version=VER_STRING_GOES_HERE
  Constant 0 : xbsIndex_r4/Constant  arith_type=Unsigned  const=0  n_bits=1  bin_pt=0  explicit_period=off  period=1  equ=P=C  opselect=C  inp2=PCIN>>17  opr=+  inp1=P  carry=CIN  dbl_ovrd=off  block_type=constant
      settings: block_version=VER_STRING_GOES_HERE
  Counter : xbsIndex_r4/Counter  cnt_type=Count Limited  cnt_to=length(coef)-1  operation=Up  start_count=0  cnt_by_val=1  arith_type=Unsigned  n_bits=ceil(log2(length(coef)))  bin_pt=0  load_pin=off  rst=off  en=off  dbl_ovrd=off  explicit_period=on  period=smpl_period/length(coef)  block_type=counter
      settings: infoedit="Configurable up, down and up/down counter.<P><P>Hardware notes: Free running counters are the least expensive in hardware.  A count limited counter is implemented by combining a counter with a comparator."  xl_area=[0, 0, 0, 0, 0, 0, 0]  block_version=VER_STRING_GOES_HERE
  Down Sample1 : xbsIndex_r4/Down Sample  sample_ratio=length(coef)  sample_phase="Last Value of Frame  (most efficient)"  en=off  latency=1  dbl_ovrd=off  block_type=dsamp
      settings: xl_area=[0, 0, 0, 0, 0, 0, 0]  block_version=VER_STRING_GOES_HERE
  MAC Engine : Subsystem
  Relational1 : xbsIndex_r4/Relational  mode=a=b  en=off  latency=3  dbl_ovrd=off  block_type=relational
      settings: xl_area=[0, 0, 0, 0, 0, 0, 0]  block_version=VER_STRING_GOES_HERE
  r0 : xbsIndex_r4/Delay  en=off  latency=2  dbl_ovrd=off  reg_retiming=off  block_type=delay
      settings: infoedit="Delay line having  configurable length.<P><P>Hardware notes: A delay line is a chain, each link of which is an SRL16 followed by a flip-flop. If register retiming is enabled, the delay line is a chain of flip-flops."  xl_area=[0, 0, 0, 0, 0, 0, 0]  block_version=VER_STRING_GOES_HERE
  r1 : xbsIndex_r4/Delay  en=off  latency=1  dbl_ovrd=off  reg_retiming=off  block_type=delay
      settings: infoedit="Delay line having  configurable length.<P><P>Hardware notes: A delay line is a chain, each link of which is an SRL16 followed by a flip-flop. If register retiming is enabled, the delay line is a chain of flip-flops."  xl_area=[0, 0, 0, 0, 0, 0, 0]  block_version=VER_STRING_GOES_HERE
  r2 : xbsIndex_r4/Delay  en=off  latency=1  dbl_ovrd=off  reg_retiming=off  block_type=delay
      settings: infoedit="Delay line having  configurable length.<P><P>Hardware notes: A delay line is a chain, each link of which is an SRL16 followed by a flip-flop. If register retiming is enabled, the delay line is a chain of flip-flops."  xl_area=[0, 0, 0, 0, 0, 0, 0]  block_version=VER_STRING_GOES_HERE
  r3 : xbsIndex_r4/Delay  en=off  latency=1  dbl_ovrd=off  reg_retiming=off  block_type=delay
      settings: infoedit="Delay line having  configurable length.<P><P>Hardware notes: A delay line is a chain, each link of which is an SRL16 followed by a flip-flop. If register retiming is enabled, the delay line is a chain of flip-flops."  xl_area=[0, 0, 0, 0, 0, 0, 0]  block_version=VER_STRING_GOES_HERE
  dout : Outport  OutDataType=sfix(16)  OutScaling=2^0
  wires:
  din/1 -> r3/1
  r1/1 -> MAC Engine/2(b)
  r0/1 -> MAC Engine/1(a)
  ASR/1 -> r0/1
  Counter/1 -> Coefficient ROM/1, ASR/2, Relational1/1
  r3/1 -> ASR/1
  Constant 0/1 -> Relational1/2
  Coefficient ROM/1 -> r1/1
  MAC Engine/1(q) -> Capture Register/1
  Down Sample1/1 -> dout/1
  Capture Register/1 -> Down Sample1/1
  Relational1/1 -> r2/1
  r2/1 -> Capture Register/2, MAC Engine/3(rst)

== system xrbsDSP_r4/2 Channel  Decimate by 2  MAC FIR Filter/2 Channel Accum ==
  d : Inport  OutDataType=sfix(16)  OutScaling=2^0
  rst : Inport  Port=2  OutDataType=sfix(16)  OutScaling=2^0
  AddSub : xbsIndex_r4/AddSub  mode=Addition  use_carryin=off  use_carryout=off  en=off  latency=0  precision=User Defined  arith_type="Signed  (2's comp)"  n_bits=ceil(log2(coef_sum*(2^(bit_width-1))))+1  bin_pt=coef_bin_pt+bin_pt  quantization=Truncate  overflow=Wrap  dbl_ovrd=off  use_behavioral_HDL=on  pipelined=off  use_rpm=off  block_type=addsub
      settings: xl_area=[18 0 0 36 0 0 0]  block_version=VER_STRING_GOES_HERE
  Delay : xbsIndex_r4/Delay  Orientation=left  en=off  latency=1  dbl_ovrd=off  reg_retiming=off  block_type=delay
      settings: infoedit="Delay line having  configurable length.<P><P>Hardware notes: A delay line is a chain, each link of which is an SRL16 followed by a flip-flop. If register retiming is enabled, the delay line is a chain of flip-flops."  xl_area=[18 36 0 0 0 0 0]  block_version=VER_STRING_GOES_HERE
  Mux : xbsIndex_r4/Mux  inputs=2  en=off  latency=0  precision=Full  arith_type="Signed  (2's comp)"  n_bits=8  bin_pt=2  quantization=Truncate  overflow=Wrap  dbl_ovrd=off  block_type=mux
      settings: infoedit=Binary points are aligned automatically.<P><P>Hardware notes: A multiplexer using tristate buffers requires fewer lookup tables but is slower.  xl_area=[36 0 0 36 0 0 0]  block_version=VER_STRING_GOES_HERE
  Register : xbsIndex_r4/Register  init=0  rst=off  en=off  dbl_ovrd=off  block_type=register
      settings: infoedit=Delay of one sample period. <P><P>Hardware notes: Implemented using flip-flops.  xl_area=[18 36 0 0 0 0 0]  block_version=VER_STRING_GOES_HERE
  q : Outport  OutDataType=sfix(16)  OutScaling=2^0
  wires:
  Delay/1 -> AddSub/2
  Register/1 -> q/1, Delay/1
  Mux/1 -> Register/1
  AddSub/1 -> Mux/3
  rst/1 -> Mux/1
  d/1 -> Mux/2, AddSub/1

== system xrbsDSP_r4/2 Channel  Decimate by 2  MAC FIR Filter/2:1 Mux ==
  din1 : Inport  OutDataType=sfix(16)  OutScaling=2^0
  din2 : Inport  Port=2  OutDataType=sfix(16)  OutScaling=2^0
  Counter : xbsIndex_r4/Counter  cnt_type=Free Running  cnt_to=Inf  operation=Up  start_count=0  cnt_by_val=1  arith_type=Unsigned  n_bits=1  bin_pt=0  load_pin=off  rst=off  en=off  dbl_ovrd=off  explicit_period=off  period=Ts/2  block_type=counter
      settings: infoedit="Configurable up, down and up/down counter.<P><P>Hardware notes: Free running counters are the least expensive in hardware.  A count limited counter is implemented by combining a counter with a comparator."  xl_area=[2 1 0 1 0 0 0]  block_version=VER_STRING_GOES_HERE
  Delay2 : xbsIndex_r4/Delay  en=off  latency=1  dbl_ovrd=off  reg_retiming=off  block_type=delay
      settings: infoedit="Delay line having  configurable length.<P><P>Hardware notes: A delay line is a chain, each link of which is an SRL16 followed by a flip-flop. If register retiming is enabled, the delay line is a chain of flip-flops."  xl_area=[0, 0, 0, 0, 0, 0, 0]  block_version=VER_STRING_GOES_HERE
  Mux : xbsIndex_r4/Mux  inputs=2  en=off  latency=0  precision=Full  arith_type="Signed  (2's comp)"  n_bits=8  bin_pt=2  quantization=Truncate  overflow=Wrap  dbl_ovrd=off  block_type=mux
      settings: infoedit=Binary points are aligned automatically.<P><P>Hardware notes: A multiplexer using tristate buffers requires fewer lookup tables but is slower.  xl_area=[0, 0, 0, 0, 0, 0, 0]  block_version=VER_STRING_GOES_HERE
  Up Sample : xbsIndex_r4/Up Sample  sample_ratio=2  copy_samples=on  dbl_ovrd=off  block_type=usamp
      settings: infoedit="Up samples input data.  Inserted values  can be zeros or copies of the most recent input sample.<P><P>Hardware notes: No hardware is needed if inserted values are copies of the input sample; otherwise, a mux and single bit flip-flop are used."  xl_area=[0, 0, 0, 0, 0, 0, 0]  block_version=VER_STRING_GOES_HERE
  Up Sample1 : xbsIndex_r4/Up Sample  sample_ratio=2  copy_samples=on  dbl_ovrd=off  block_type=usamp
      settings: infoedit="Up samples input data.  Inserted values  can be zeros or copies of the most recent input sample.<P><P>Hardware notes: No hardware is needed if inserted values are copies of the input sample; otherwise, a mux and single bit flip-flop are used."  xl_area=[0, 0, 0, 0, 0, 0, 0]  block_version=VER_STRING_GOES_HERE
  Up Sample2 : xbsIndex_r4/Up Sample  sample_ratio=length(coef)/4  copy_samples=on  dbl_ovrd=off  block_type=usamp
      settings: infoedit="Up samples input data.  Inserted values  can be zeros or copies of the most recent input sample.<P><P>Hardware notes: No hardware is needed if inserted values are copies of the input sample; otherwise, a mux and single bit flip-flop are used."  xl_area=[0, 0, 0, 0, 0, 0, 0]  block_version=VER_STRING_GOES_HERE
  dout : Outport  OutDataType=sfix(16)  OutScaling=2^0
  wires:
  Up Sample2/1 -> dout/1
  din2/1 -> Up Sample1/1
  din1/1 -> Up Sample/1
  Delay2/1 -> Up Sample2/1
  Mux/1 -> Delay2/1
  Counter/1 -> Mux/1
  Up Sample1/1 -> Mux/3
  Up Sample/1 -> Mux/2

== system xrbsDSP_r4/2 Channel  Decimate by 2  MAC FIR Filter/Accum Control ==
  Constant1 : xbsIndex_r4/Constant  arith_type=Unsigned  const=2  n_bits=2  bin_pt=0  explicit_period=off  period=1  equ=P=C  opselect=C  inp2=PCIN>>17  opr=+  inp1=P  carry=CIN  dbl_ovrd=off  block_type=constant
      settings: block_version=VER_STRING_GOES_HERE
  Constant4 : xbsIndex_r4/Constant  arith_type=Unsigned  const=0  n_bits=2  bin_pt=0  explicit_period=off  period=1  equ=P=C  opselect=C  inp2=PCIN>>17  opr=+  inp1=P  carry=CIN  dbl_ovrd=off  block_type=constant
      settings: block_version=VER_STRING_GOES_HERE
  Constant5 : xbsIndex_r4/Constant  arith_type=Unsigned  const=1  n_bits=2  bin_pt=0  explicit_period=off  period=1  equ=P=C  opselect=C  inp2=PCIN>>17  opr=+  inp1=P  carry=CIN  dbl_ovrd=off  block_type=constant
      settings: block_version=VER_STRING_GOES_HERE
  Counter : xbsIndex_r4/Counter  cnt_type=Free Running  cnt_to=Inf  operation=Up  start_count=0  cnt_by_val=1  arith_type=Unsigned  n_bits=2  bin_pt=0  load_pin=off  rst=off  en=off  dbl_ovrd=off  explicit_period=off  period=Ts/2  block_type=counter
      settings: infoedit="Configurable up, down and up/down counter.<P><P>Hardware notes: Free running counters are the least expensive in hardware.  A count limited counter is implemented by combining a counter with a comparator."  xl_area=[1 2 0 2 0 0 0]  block_version=VER_STRING_GOES_HERE
  Logical : xbsIndex_r4/Logical  logical_function=OR  inputs=2  en=off  latency=0  precision=Full  arith_type=Unsigned  n_bits=8  bin_pt=2  quantization=Truncate  overflow=Wrap  align_bp=on  dbl_ovrd=off  block_type=logical
      settings: xl_area=[1 0 0 1 0 0 0]  block_version=VER_STRING_GOES_HERE
  Relational1 : xbsIndex_r4/Relational  mode=a=b  en=off  latency=0  dbl_ovrd=off  block_type=relational
      settings: xl_area=[2 0 0 1 0 0 0]  block_version=VER_STRING_GOES_HERE
  Relational4 : xbsIndex_r4/Relational  mode=a=b  en=off  latency=0  dbl_ovrd=off  block_type=relational
      settings: xl_area=[2 0 0 1 0 0 0]  block_version=VER_STRING_GOES_HERE
  Relational5 : xbsIndex_r4/Relational  mode=a=b  en=off  latency=0  dbl_ovrd=off  block_type=relational
      settings: xl_area=[2 0 0 1 0 0 0]  block_version=VER_STRING_GOES_HERE
  rst : Outport  OutDataType=sfix(16)  OutScaling=2^0
  en_a : Outport  Port=2  OutDataType=sfix(16)  OutScaling=2^0
  en_b : Outport  Port=3  OutDataType=sfix(16)  OutScaling=2^0
  wires:
  Relational1/1 -> en_b/1
  Constant1/1 -> Relational1/2
  Logical/1 -> rst/1
  Relational5/1 -> en_a/1, Logical/2
  Relational4/1 -> Logical/1
  Constant5/1 -> Relational5/2
  Constant4/1 -> Relational4/2
  Counter/1 -> Relational4/1, Relational1/1, Relational5/1

== system xrbsDSP_r4/2 Channel  Decimate by 2  MAC FIR Filter/Data Buffer ==
  din : Inport  OutDataType=sfix(16)  OutScaling=2^0
  data_addr : Inport  Port=2  OutDataType=sfix(16)  OutScaling=2^0
  en : Inport  Port=3  OutDataType=sfix(16)  OutScaling=2^0
  coef_addr : Inport  Port=4  OutDataType=sfix(16)  OutScaling=2^0
  ASR : xbsIndex_r4/Addressable Shift Register  infer_latency=on  depth=2  initVector=[0]  en=on  dbl_ovrd=off  use_behavioral_HDL=off  use_rpm=off  block_type=addrsr
      settings: infoedit="Delay of configurable length.  Any element in the delay line can be addressed and driven onto the output port.<P><P>Hardware notes: Implemented using SRL16s.  If a Virtex-II device is used, multiple SRLC16s are cascaded together."  xl_area=[0, 0, 0, 0, 0, 0, 0]  block_version=VER_STRING_GOES_HERE
  Delay1 : xbsIndex_r4/Delay  en=off  latency=1  dbl_ovrd=off  reg_retiming=off  block_type=delay
      settings: infoedit="Delay line having  configurable length.<P><P>Hardware notes: A delay line is a chain, each link of which is an SRL16 followed by a flip-flop. If register retiming is enabled, the delay line is a chain of flip-flops."  xl_area=[0, 0, 0, 0, 0, 0, 0]  block_version=VER_STRING_GOES_HERE
  ROM : xbsIndex_r4/ROM  depth=length(coef)  initVector=coef  rst=off  init_reg=0  en=off  latency=1  arith_type="Signed  (2's comp)"  n_bits=coef_bit_width  bin_pt=coef_bin_pt  dbl_ovrd=off  distributed_mem=Block RAM  use_rpm=off  block_type=sprom
      settings: xl_area=[0, 0, 0, 0, 0, 0, 0]  block_version=VER_STRING_GOES_HERE
  dout : Outport  OutDataType=sfix(16)  OutScaling=2^0
  coef_out : Outport  Port=2  OutDataType=sfix(16)  OutScaling=2^0
  wires:
  Delay1/1 -> dout/1
  ROM/1 -> coef_out/1
  coef_addr/1 -> ROM/1
  ASR/1 -> Delay1/1
  data_addr/1 -> ASR/2
  din/1 -> ASR/1
  en/1 -> ASR/3

== system xrbsDSP_r4/2 Channel  Decimate by 2  MAC FIR Filter/Memory Control ==
  Addr Counter : xbsIndex_r4/Counter  cnt_type=Count Limited  cnt_to=length(coef)-4  operation=Up  start_count=0  cnt_by_val=4  arith_type=Unsigned  n_bits=ceil(log2(length(coef)-1))  bin_pt=0  load_pin=off  rst=off  en=off  dbl_ovrd=off  explicit_period=off  period=Ts/(length(coef)/2)  block_type=counter
      settings: infoedit="Configurable up, down and up/down counter.<P><P>Hardware notes: Free running counters are the least expensive in hardware.  A count limited counter is implemented by combining a counter with a comparator."  xl_area=[0, 0, 0, 0, 0, 0, 0]  block_version=VER_STRING_GOES_HERE
  Coef Counter : xbsIndex_r4/Counter  cnt_type=Count Limited  cnt_to=length(coef)-1  operation=Up  start_count=0  cnt_by_val=1  arith_type=Unsigned  n_bits=ceil(log2(length(coef)-1))  bin_pt=0  load_pin=off  rst=off  en=off  dbl_ovrd=off  explicit_period=off  period=Ts/(length(coef)/2)  block_type=counter
      settings: infoedit="Configurable up, down and up/down counter.<P><P>Hardware notes: Free running counters are the least expensive in hardware.  A count limited counter is implemented by combining a counter with a comparator."  xl_area=[0, 0, 0, 0, 0, 0, 0]  block_version=VER_STRING_GOES_HERE
  Constant : xbsIndex_r4/Constant  arith_type=Unsigned  const=length(coef)-4  n_bits=ceil(log2(length(coef)-4))  bin_pt=0  explicit_period=off  period=1  equ=P=C  opselect=C  inp2=PCIN>>17  opr=+  inp1=P  carry=CIN  dbl_ovrd=off  block_type=constant
      settings: block_version=VER_STRING_GOES_HERE
  Relational : xbsIndex_r4/Relational  mode=a=b  en=off  latency=0  dbl_ovrd=off  block_type=relational
      settings: xl_area=[0, 0, 0, 0, 0, 0, 0]  block_version=VER_STRING_GOES_HERE
  data_addr : Outport  OutDataType=sfix(16)  OutScaling=2^0
  we : Outport  Port=2  OutDataType=sfix(16)  OutScaling=2^0
  coef_addr : Outport  Port=3  OutDataType=sfix(16)  OutScaling=2^0
  wires:
  Coef Counter/1 -> coef_addr/1
  Relational/1 -> we/1
  Constant/1 -> Relational/2
  Addr Counter/1 -> data_addr/1, Relational/1
